simulink model "ejemplo01"  (R2021b)
settings: Solver=VariableStepAuto  StartTime=0.0  StopTime=10.0  RelTol=1e-3
settings Model: Creator=juandiegocastropadilla  LastModifiedBy=juandiegocastropadilla

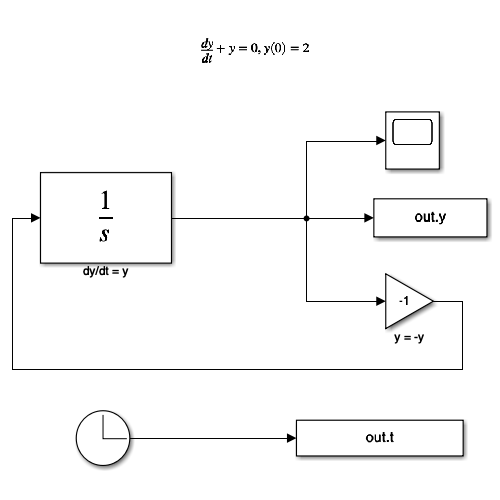
[thumbnail: Simulink's stored preview of the top-level diagram]
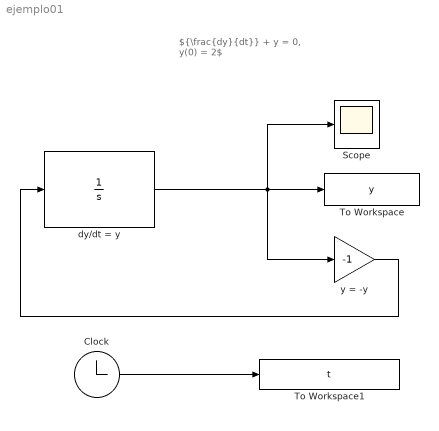
== system ejemplo01 ==
  note: ${\frac{dy}{dt}} + y = 0, y(0) = 2$
  Clock : Clock
  Scope : Scope
  To Workspace : ToWorkspace  VariableName=y  SampleTime=-1
  To Workspace1 : ToWorkspace  VariableName=t  SampleTime=-1
  dy/dt = y : Integrator  InitialCondition=2
  y = -y : Gain  Gain=-1
  wires:
  dy/dt = y/1 -> y = -y/1, To Workspace/1, Scope/1
  y = -y/1 -> dy/dt = y/1
  Clock/1 -> To Workspace1/1
